simulink model "sim_DF_fixp16_alu"  (R2020b)
settings: Solver=FixedStepDiscrete  StartTime=0.0  StopTime=0.8  FixedStep=DSPBASampleTime  RelTol=1e-3  EnableMultiTasking=on
PreLoadFcn:
  | setup_sim_DF_fixp16_alu;
InitFcn:
  | setup_sim_DF_fixp16_alu;
values from neighbouring files (symbols this model uses):
  ClockFrequency = 100    [setup_DF_fixp16_alu_av.m]    (also in setup_sim_DF_fixp16_alu.m; setup_verify_DF_fixp16_alu.m)
  DSPBASampleTime = FoldingFactor / (ClockFrequency * 1e6)    (= 5e-06)    [setup_DF_fixp16_alu_av.m]    (also in setup_sim_DF_fixp16_alu.m; setup_verify_DF_fixp16_alu.m)
  FoldingFactor = 500    [setup_DF_fixp16_alu_av.m]    (also in setup_sim_DF_fixp16_alu.m; setup_verify_DF_fixp16_alu.m)
  PwmMax = 9375    [setup_sim_DF_fixp16_alu.m]    (also in setup_verify_DF_fixp16_alu.m)
undefined symbols (not defined in the file or in its folder): DiscIntNeverNeededParam, I_max, Position_PI_Limit
libraries: simulink x8, DSPBABase x7, foc_blocks x2
settings Model: Creator=tchau  LastModifiedBy=mhonman
settings DataIOCC: SaveFormat=Array  SaveOutput=off  SignalLogging=off  DSMLogging=off  SaveTime=off  ReturnWorkspaceOutputs=off
settings OptimizationCC: BlockReduction=off  ConditionallyExecuteInputs=off  DefaultParameterBehavior=Inlined  InlineInvariantSignals=on  EfficientFloat2IntCast=on  LifeSpan=inf  SimCompilerOptimization=on
settings DebuggingCC: AlgebraicLoopMsg=error  SolverPrmCheckMsg=warning  SingleTaskRateTransMsg=error  SFUnexpectedBacktrackingDiag=warning  SFNoUnconditionalDefaultTransitionDiag=warning  SFExecutionAtInitializationDiag=none  ArithmeticOperatorsInVariantConditions=warning
settings HardwareCC: ProdBitPerPointer=32  ProdBitPerSizeT=32  ProdBitPerPtrDiffT=32  ProdLargestAtomicFloat=None  ProdIntDivRoundTo=Undefined  ProdEndianess=Unspecified  ProdWordSize=32  ProdHWDeviceType=ASIC/FPGA->ASIC/FPGA  TargetBitPerLong=64  TargetBitPerPointer=64  TargetBitPerSizeT=64  TargetBitPerPtrDiffT=64  TargetLongLongMode=on  TargetIntDivRoundTo=Zero  TargetEndianess=LittleEndian  TargetWordSize=64  TargetHWDeviceType=MATLAB Host  ProdEqTarget=off
settings ModelReferenceCC: PropagateSignalLabelsOutOfModel=off
settings SFSimCC: SimUseLocalCustomCode=off  CustomCodeUndefinedFunction=UseInterfaceOnly
settings RTWCC: RTWUseLocalCustomCode=off
settings CodeAppCC: StateflowObjectComments=on
settings GRTTargetCC: TargetLangStandard=C89/C90 (ANSI)  MatFileLogging=off  SupportNonFinite=off
settings ConfigComp: CovMetricSettings=dw  CovSaveCumulativeToWorkspaceVar=on  CovSaveSingleToWorkspaceVar=on  CovExternalEMLEnable=off

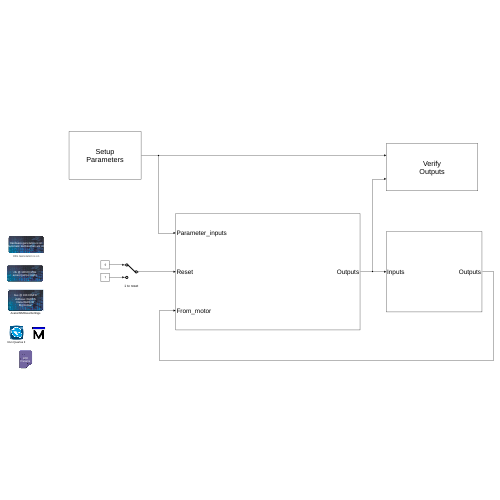
[thumbnail: Simulink's stored preview of the top-level diagram]
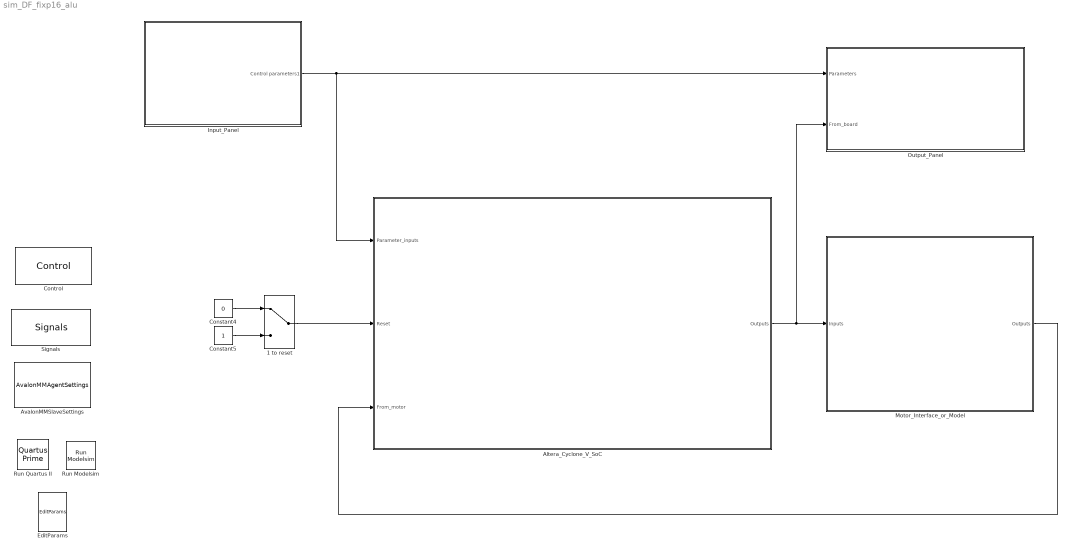
== system sim_DF_fixp16_alu ==
  1 to reset : ManualSwitch
  Altera_Cyclone_V_SoC : Subsystem
  AvalonMMSlaveSettings : DSPBABase/AvalonMMAgentSettings
  Constant4 : Constant  Value=0  OutDataTypeStr=boolean
  Constant5 : Constant  OutDataTypeStr=boolean
  Control : DSPBABase/Control  generate=on  language=VHDL  destination=./rtlmax10  destination_gui=./rtlmax10  make_full_path=off  path_is_relative=on  autotestbench=on  signaldepth=2  coveragetestbench=off  logs=off  spacewidth=2  spacenum=1  addrwidth=6  datawidth=32  dataendian=Big Endian  hierarchicalnames=off  ramThresholdBits=-1  distRamThresholdBits=-1  mlabThresholdBits=-1  hardMultiplierThresholdLuts=-1  version=20090407  errorOnChanMismatch=1  errorOnGPIOMismatch=0  importModelsimResults=0  cycleAccurate=off  reinterpretCastMult=off  paramFile=osim_DF_fixp16_alu_params.xml
      settings: AttributesFormatString=HDL Generation is %<generate>
  EditParams : DSPBABase/EditParams  version=20090407
  Input_Panel : Subsystem
      mask Display: fprintf('Setup\nParameters')
  Motor_Interface_or_Model : Subsystem
  Output_Panel : Subsystem
      mask Display: fprintf('Verify\nOutputs')
  Run Modelsim : DSPBABase/Run Modelsim  version=20090407
  Run Quartus II : DSPBABase/Quartus Prime  version=20090407
  Signals : DSPBABase/Signals  clk=clk  freq=ClockFrequency  margin=0  rst=areset  rstactive=High  bus=bus  enbusclock=off  busfreq=100  bussync=on  version=20090407
  wires:
  Input_Panel/1(Control parameters1) -> Altera_Cyclone_V_SoC/1(Parameter_inputs), Output_Panel/1(Parameters)
  Constant4/1 -> 1 to reset/1
  Constant5/1 -> 1 to reset/2
  1 to reset/1 -> Altera_Cyclone_V_SoC/2(Reset)
  Altera_Cyclone_V_SoC/1(Outputs) -> Motor_Interface_or_Model/1(Inputs), Output_Panel/2(From_board)
  Motor_Interface_or_Model/1(Outputs) -> Altera_Cyclone_V_SoC/3(From_motor)

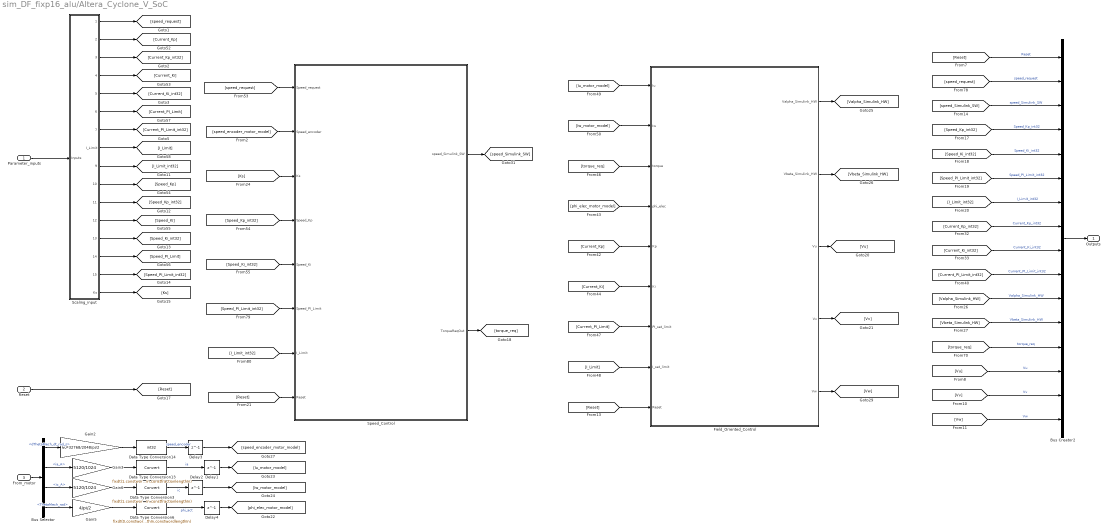
== system sim_DF_fixp16_alu/Altera_Cyclone_V_SoC ==
  Parameter_inputs : Inport
  Reset : Inport  Port=2  PortDimensions=1
  From_motor : Inport  Port=3
  Bus Creator2 : BusCreator  Inputs=16
  Bus Selector : BusSelector  OutputSignals=dThetaMech_dt_rad_s,ia_A,ic_A,ThetaMech_rad
  Data Type Conversion13 : DataTypeConversion  OutDataTypeStr=fixdt(1,constwordlengthIn,constfractionlengthIn)
  Data Type Conversion14 : DataTypeConversion  OutDataTypeStr=int32
  Data Type Conversion3 : DataTypeConversion  OutDataTypeStr=fixdt(1,constwordlengthIn,constfractionlengthIn)
  Data Type Conversion6 : DataTypeConversion  OutDataTypeStr=fixdt(0,constwordlengthIn,constwordlengthIn)
  Delay{1..4} (4 alike) : Delay  DelayLength=1  InitialCondition=0
  Field_Oriented_Control : Subsystem
      mask Display: fprintf('Field-Oriented\nControl')
  Gain2 : Gain  Gain=60*32768/2048/pi/2  OutDataTypeStr=single
  Gain3 : Gain  Gain=5120/1024  OutDataTypeStr=single
  Gain5 : Gain  Gain=4/pi/2  OutDataTypeStr=single
  Gain6 : Gain  Gain=5120/1024  OutDataTypeStr=single
  Scaling_input : Subsystem
  Speed_Control : Subsystem
      mask Display: fprintf('Speed\nControl')
  Outputs : Outport
  wires:
  Speed_Control/2(TorqueReqOut) -> [torque_req]
  Speed_Control/1(speed_Simulink_SW) -> [speed_Simulink_SW]
  [Reset] -> Speed_Control/8(Reset)
  [Ks] -> Speed_Control/3(Ks)
  [speed_Simulink_SW] -> Bus Creator2/3  "speed_Simulink_SW"
  Reset/1 -> [Reset]
  [speed_request] -> Bus Creator2/2  "speed_request"
  Parameter_inputs/1 -> Scaling_input/1(Inputs)
  Scaling_input/1(speed_request) -> [speed_request]
  Scaling_input/2(Current_Kp) -> [Current_Kp]
  Scaling_input/3(Current_Kp_int32) -> [Current_Kp_int32]
  Scaling_input/4(Current_Ki) -> [Current_Ki]
  Scaling_input/5(Current_Ki_int32) -> [Current_Ki_int32]
  Scaling_input/6(Current_PI_Limit) -> [Current_PI_Limit]
  Scaling_input/7(Current_PI_Limit_int32) -> [Current_PI_Limit_int32]
  Scaling_input/8(I_Limit) -> [I_Limit]
  Scaling_input/9(I_Limit_int32) -> [I_Limit_int32]
  Scaling_input/10(Speed_Kp) -> [Speed_Kp]
  Scaling_input/11(Speed_Kp_int32) -> [Speed_Kp_int32]
  Scaling_input/12(Speed_Ki) -> [Speed_Ki]
  Scaling_input/13(Speed_Ki_int32) -> [Speed_Ki_int32]
  Scaling_input/14(Speed_PI_Limit) -> [Speed_PI_Limit]
  Scaling_input/15(Speed_PI_Limit_int32) -> [Speed_PI_Limit_int32]
  Scaling_input/16(Ks) -> [Ks]
  [speed_request] -> Speed_Control/1(Speed_request)
  [Speed_Kp_int32] -> Speed_Control/4(Speed_Kp)
  [Speed_Ki_int32] -> Speed_Control/5(Speed_Ki)
  [Speed_PI_Limit_int32] -> Speed_Control/6(Speed_PI_Limit)
  [I_Limit_int32] -> Speed_Control/7(I_Limit)
  [Speed_Kp_int32] -> Bus Creator2/4  "Speed_Kp_int32"
  [Speed_Ki_int32] -> Bus Creator2/5  "Speed_Ki_int32"
  [Speed_PI_Limit_int32] -> Bus Creator2/6  "Speed_PI_Limit_int32"
  [I_Limit_int32] -> Bus Creator2/7  "I_Limit_int32"
  [Current_Kp_int32] -> Bus Creator2/8  "Current_Kp_int32"
  [Current_Ki_int32] -> Bus Creator2/9  "Current_Ki_int32"
  [Current_PI_Limit_int32] -> Bus Creator2/10  "Current_PI_Limit_int32"
  [Reset] -> Bus Creator2/1  "Reset"
  Bus Creator2/1 -> Outputs/1
  [Valpha_Simulink_HW] -> Bus Creator2/11  "Valpha_Simulink_HW"
  [Vbeta_Simulink_HW] -> Bus Creator2/12  "Vbeta_Simulink_HW"
  [torque_req] -> Bus Creator2/13  "torque_req"
  [Iu_motor_model] -> Field_Oriented_Control/1(Iu)
  [Iw_motor_model] -> Field_Oriented_Control/2(Iw)
  [torque_req] -> Field_Oriented_Control/3(torque)
  [phi_elec_motor_model] -> Field_Oriented_Control/4(phi_elec)
  [Current_Kp] -> Field_Oriented_Control/5(Kp)
  [Current_Ki] -> Field_Oriented_Control/6(Ki)
  [Current_PI_Limit] -> Field_Oriented_Control/7(PI_sat_limit)
  [I_Limit] -> Field_Oriented_Control/8(I_sat_limit)
  [Reset] -> Field_Oriented_Control/9(Reset)
  Field_Oriented_Control/1(Valpha_Simulink_HW) -> [Valpha_Simulink_HW]
  Field_Oriented_Control/2(Vbeta_Simulink_HW) -> [Vbeta_Simulink_HW]
  Field_Oriented_Control/3(Vu) -> [Vu]
  From_motor/1 -> Bus Selector/1
  [speed_encoder_motor_model] -> Speed_Control/2(Speed_encoder)
  Delay1/1 -> [Iu_motor_model]
  Delay2/1 -> [Iw_motor_model]
  Delay4/1 -> [phi_elec_motor_model]
  Bus Selector/3 -> Gain6/1  "<ic_A>"
  Delay3/1 -> [speed_encoder_motor_model]
  Bus Selector/1 -> Gain2/1  "<dThetaMech_dt_rad_s>"
  Bus Selector/4 -> Gain5/1  "<ThetaMech_rad>"
  Bus Selector/2 -> Gain3/1  "<ia_A>"
  [Vu] -> Bus Creator2/14  "Vu"
  [Vv] -> Bus Creator2/15  "Vv"
  [Vw] -> Bus Creator2/16  "Vw"
  Gain2/1 -> Data Type Conversion14/1
  Data Type Conversion14/1 -> Delay3/1  "speed_encoder"
  Gain5/1 -> Data Type Conversion6/1
  Data Type Conversion6/1 -> Delay4/1  "phi_act"
  Gain3/1 -> Data Type Conversion13/1
  Data Type Conversion13/1 -> Delay1/1  "ia"
  Gain6/1 -> Data Type Conversion3/1
  Data Type Conversion3/1 -> Delay2/1  "ic"
  Field_Oriented_Control/4(Vv) -> [Vv]
  Field_Oriented_Control/5(Vw) -> [Vw]

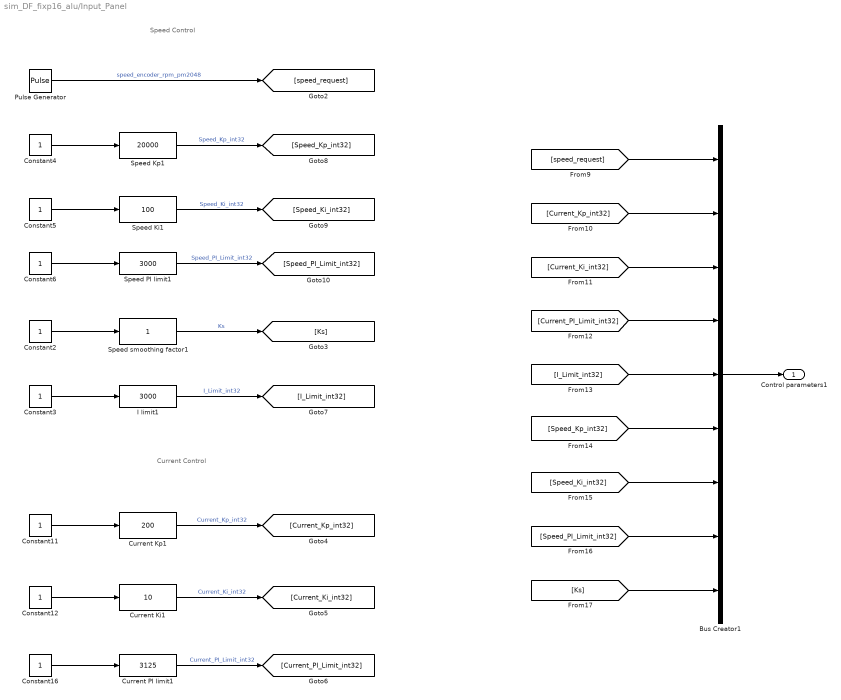
== system sim_DF_fixp16_alu/Input_Panel ==
  note: Speed Control
  note: Current Control
  Bus Creator1 : BusCreator  Inputs=9
  Constant{3..6,11..12,16} (7 alike) : Constant  OutDataTypeStr=int32
  Constant2 : Constant  OutDataTypeStr=fixdt(0,16,15)
  Current Ki1 : simulink/Math Operations/Slider Gain  gain=10  low=0  high=100
  Current Kp1 : simulink/Math Operations/Slider Gain  gain=200  low=0  high=1000
  Current PI limit1 : simulink/Math Operations/Slider Gain  gain=3125  low=0  high=10000
  I limit1 : simulink/Math Operations/Slider Gain  gain=3000  low=0  high=10000
  Pulse Generator : DiscretePulseGenerator  Amplitude=50  Period=ClockFrequency * 1e6 / FoldingFactor * 5  PulseWidth=ClockFrequency * 1e6 / FoldingFactor * 2.5  SampleTime=DSPBASampleTime
  Speed Ki1 : simulink/Math Operations/Slider Gain  gain=100  low=0  high=1000
  Speed Kp1 : simulink/Math Operations/Slider Gain  gain=20000  low=0  high=100000
  Speed PI limit1 : simulink/Math Operations/Slider Gain  gain=3000  low=0  high=10000
  Speed smoothing factor1 : simulink/Math Operations/Slider Gain  gain=1  low=0  high=1
  Control parameters1 : Outport
  wires:
  Pulse Generator/1 -> [speed_request]  "speed_encoder_rpm_pm2048"
  [Ks] -> Bus Creator1/9
  [Speed_PI_Limit_int32] -> Bus Creator1/8
  [Speed_Ki_int32] -> Bus Creator1/7
  [Speed_Kp_int32] -> Bus Creator1/6
  [I_Limit_int32] -> Bus Creator1/5
  [Current_PI_Limit_int32] -> Bus Creator1/4
  [Current_Ki_int32] -> Bus Creator1/3
  [Current_Kp_int32] -> Bus Creator1/2
  [speed_request] -> Bus Creator1/1
  Bus Creator1/1 -> Control parameters1/1
  Constant2/1 -> Speed smoothing factor1/1
  Speed smoothing factor1/1 -> [Ks]  "Ks"
  Speed Kp1/1 -> [Speed_Kp_int32]  "Speed_Kp_int32"
  Speed Ki1/1 -> [Speed_Ki_int32]  "Speed_Ki_int32"
  Speed PI limit1/1 -> [Speed_PI_Limit_int32]  "Speed_PI_Limit_int32"
  Constant4/1 -> Speed Kp1/1
  Constant5/1 -> Speed Ki1/1
  Constant6/1 -> Speed PI limit1/1
  Current Kp1/1 -> [Current_Kp_int32]  "Current_Kp_int32"
  Current Ki1/1 -> [Current_Ki_int32]  "Current_Ki_int32"
  Current PI limit1/1 -> [Current_PI_Limit_int32]  "Current_PI_Limit_int32"
  I limit1/1 -> [I_Limit_int32]  "I_Limit_int32"
  Constant11/1 -> Current Kp1/1
  Constant12/1 -> Current Ki1/1
  Constant16/1 -> Current PI limit1/1
  Constant3/1 -> I limit1/1

== system sim_DF_fixp16_alu/Motor_Interface_or_Model ==
  Inputs : Inport
  Bus Selector : BusSelector  OutputSignals=Vu,Vv,Vw
  Constant1 : Constant  Value=0  OutDataTypeStr=Inherit: Inherit via back propagation
  Data Type Conversion1 : DataTypeConversion  OutDataTypeStr=double
  Data Type Conversion4 : DataTypeConversion  OutDataTypeStr=double
  Data Type Conversion5 : DataTypeConversion  OutDataTypeStr=double
  MotorContinuousTime4 : Subsystem  mask(AlteraPMSM){R_ohm=21.4/2, L_H=37.5e-3/2, Ke_Vs_rad=0.85/sqrt(2), Kt_Nm_A=0.85/sqrt(2), PolePairs_int=4, J_kgm2=0.33e-4}
      mask prompts: R_ohm "Phase resistance [Ohm]"; L_H "Phase inductance [H]"; Ke_Vs_rad "Back-emf constant kE, based on peak phase values [Vs/rad]"; Kt_Nm_A "Motor torque constant kT, based on peak phase values [Nm/A]"; PolePairs_int "Number of pole pairs (0.5*n poles)  [integer]"; J_kgm2 "Mechanical inertia [kgm^2]"
      mask help: Altera motor model
      mask Display: fprintf('Motor\nModel')
  Outputs : Outport
  wires:
  Constant1/1 -> MotorContinuousTime4/4(Load Torque [Nm])
  Inputs/1 -> Bus Selector/1
  Data Type Conversion4/1 -> MotorContinuousTime4/1(Va_V)
  Data Type Conversion1/1 -> MotorContinuousTime4/2(Vb_V)
  Data Type Conversion5/1 -> MotorContinuousTime4/3(Vc_V)
  Bus Selector/1 -> Data Type Conversion4/1  "<Vu>"
  Bus Selector/2 -> Data Type Conversion1/1  "<Vv>"
  Bus Selector/3 -> Data Type Conversion5/1  "<Vw>"
  MotorContinuousTime4/1(OutputBus) -> Outputs/1

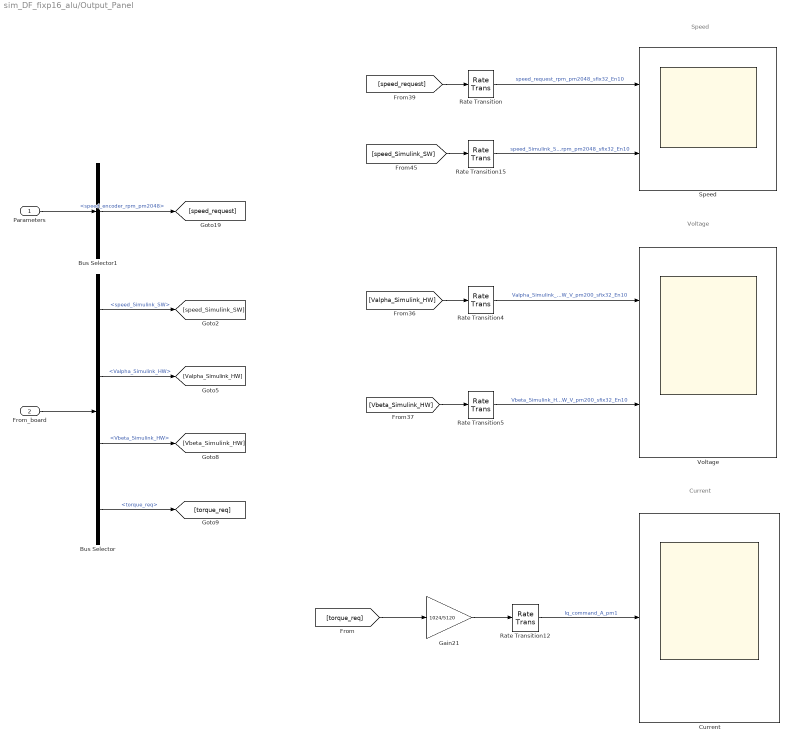
== system sim_DF_fixp16_alu/Output_Panel ==
  note: Speed
  note: Voltage
  note: Current
  Parameters : Inport
  From_board : Inport  Port=2
  Bus Selector : BusSelector  OutputSignals=speed_Simulink_SW,Valpha_Simulink_HW,Vbeta_Simulink_HW,torque_req
  Bus Selector1 : BusSelector  OutputSignals=speed_encoder_rpm_pm2048
  Current : Scope
  Gain21 : Gain  Gain=1024/5120
  Rate Transition{,4..5,12,15} (5 alike) : RateTransition
  Speed : Scope  NumInputPorts=2
  Voltage : Scope  NumInputPorts=2
  wires:
  Rate Transition4/1 -> Voltage/1  "Valpha_Simulink_HW_V_pm200_sfix32_En10"
  Rate Transition5/1 -> Voltage/2  "Vbeta_Simulink_HW_V_pm200_sfix32_En10"
  Rate Transition/1 -> Speed/1  "speed_request_rpm_pm2048_sfix32_En10"
  [speed_request] -> Rate Transition/1
  Rate Transition15/1 -> Speed/2  "speed_Simulink_SW_rpm_pm2048_sfix32_En10"
  [speed_Simulink_SW] -> Rate Transition15/1
  [torque_req] -> Gain21/1
  Rate Transition12/1 -> Current/1  "Iq_command_A_pm1"
  Gain21/1 -> Rate Transition12/1
  [Valpha_Simulink_HW] -> Rate Transition4/1
  [Vbeta_Simulink_HW] -> Rate Transition5/1
  From_board/1 -> Bus Selector/1
  Parameters/1 -> Bus Selector1/1
  Bus Selector1/1 -> [speed_request]  "<speed_encoder_rpm_pm2048>"
  Bus Selector/1 -> [speed_Simulink_SW]  "<speed_Simulink_SW>"
  Bus Selector/2 -> [Valpha_Simulink_HW]  "<Valpha_Simulink_HW>"
  Bus Selector/3 -> [Vbeta_Simulink_HW]  "<Vbeta_Simulink_HW>"
  Bus Selector/4 -> [torque_req]  "<torque_req>"

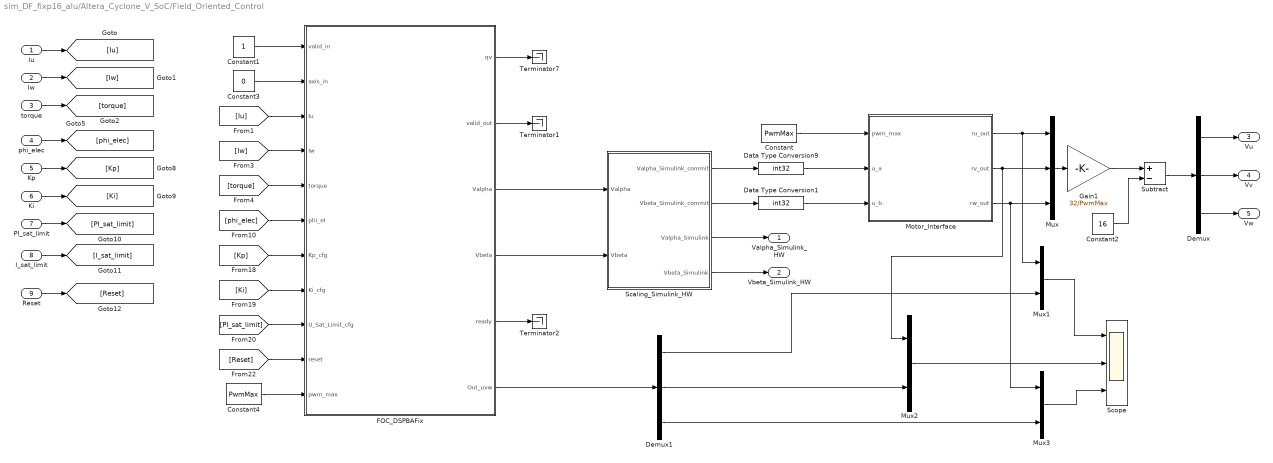
== system sim_DF_fixp16_alu/Altera_Cyclone_V_SoC/Field_Oriented_Control ==
  Iu : Inport
  Iw : Inport  Port=2
  torque : Inport  Port=3
  phi_elec : Inport  Port=4
  Kp : Inport  Port=5
  Ki : Inport  Port=6
  PI_sat_limit : Inport  Port=7
  I_sat_limit : Inport  Port=8
  Reset : Inport  Port=9
  Constant : Constant  Value=PwmMax  OutDataTypeStr=uint16
  Constant1 : Constant  OutDataTypeStr=boolean
  Constant2 : Constant  Value=16  OutDataTypeStr=int32
  Constant3 : Constant  Value=0  OutDataTypeStr=uint32
  Constant4 : Constant  Value=PwmMax  OutDataTypeStr=uint16
  Data Type Conversion1 : DataTypeConversion  OutDataTypeStr=int32
  Data Type Conversion9 : DataTypeConversion  OutDataTypeStr=int32
  Demux : Demux  Outputs=3
  Demux1 : Demux  Outputs=3
  FOC_DSPBAFix : Subsystem
  Gain1 : Gain  Gain=32/PwmMax
  Motor_Interface : MATLAB Function  TreatAsAtomicUnit=on
  Mux : Mux  Inputs=3
  Mux1 : Mux  Inputs=2
  Mux2 : Mux  Inputs=2
  Mux3 : Mux  Inputs=2
  Scaling_Simulink_HW : Subsystem
  Scope : Scope  NumInputPorts=3
  Subtract : Sum  Inputs=+-
  Terminator1 : Terminator
  Terminator2 : Terminator
  Terminator7 : Terminator
  Valpha_Simulink_HW : Outport
  Vbeta_Simulink_HW : Outport  Port=2
  Vu : Outport  Port=3
  Vv : Outport  Port=4
  Vw : Outport  Port=5
  wires:
  FOC_DSPBAFix/3(Valpha) -> Scaling_Simulink_HW/1(Valpha)
  FOC_DSPBAFix/4(Vbeta) -> Scaling_Simulink_HW/2(Vbeta)
  Scaling_Simulink_HW/3(Valpha_Simulink) -> Valpha_Simulink_HW/1
  Scaling_Simulink_HW/4(Vbeta_Simulink) -> Vbeta_Simulink_HW/1
  Iu/1 -> [Iu]
  [Iu] -> FOC_DSPBAFix/3(Iu)
  [Iw] -> FOC_DSPBAFix/4(Iw)
  Iw/1 -> [Iw]
  torque/1 -> [torque]
  [torque] -> FOC_DSPBAFix/5(torque)
  phi_elec/1 -> [phi_elec]
  [phi_elec] -> FOC_DSPBAFix/6(phi_el)
  Kp/1 -> [Kp]
  Ki/1 -> [Ki]
  PI_sat_limit/1 -> [PI_sat_limit]
  I_sat_limit/1 -> [I_sat_limit]
  Reset/1 -> [Reset]
  [Kp] -> FOC_DSPBAFix/7(Kp_cfg)
  [Ki] -> FOC_DSPBAFix/8(Ki_cfg)
  [PI_sat_limit] -> FOC_DSPBAFix/9(U_Sat_Limit_cfg)
  [Reset] -> FOC_DSPBAFix/10(reset)
  Scaling_Simulink_HW/1(Valpha_Simulink_commit) -> Data Type Conversion9/1
  Scaling_Simulink_HW/2(Vbeta_Simulink_commit) -> Data Type Conversion1/1
  Constant1/1 -> FOC_DSPBAFix/1(valid_in)
  Constant3/1 -> FOC_DSPBAFix/2(axis_in)
  FOC_DSPBAFix/1(qv) -> Terminator7/1
  FOC_DSPBAFix/2(valid_out) -> Terminator1/1
  FOC_DSPBAFix/5(ready) -> Terminator2/1
  Constant4/1 -> FOC_DSPBAFix/11(pwm_max)
  FOC_DSPBAFix/6(Out_uvw) -> Demux1/1
  Mux2/1 -> Scope/2
  Mux1/1 -> Scope/1
  Demux1/3 -> Mux3/2
  Demux1/2 -> Mux2/2
  Mux3/1 -> Scope/3
  Demux1/1 -> Mux1/2
  Demux/2 -> Vv/1
  Mux/1 -> Gain1/1
  Demux/3 -> Vw/1
  Constant2/1 -> Subtract/2
  Motor_Interface/3(rw_out) -> Mux3/1, Mux/3
  Demux/1 -> Vu/1
  Motor_Interface/1(ru_out) -> Mux1/1, Mux/1
  Subtract/1 -> Demux/1
  Motor_Interface/2(rv_out) -> Mux2/1, Mux/2
  Gain1/1 -> Subtract/1
  Data Type Conversion1/1 -> Motor_Interface/3(u_b)
  Data Type Conversion9/1 -> Motor_Interface/2(u_a)
  Constant/1 -> Motor_Interface/1(pwm_max)

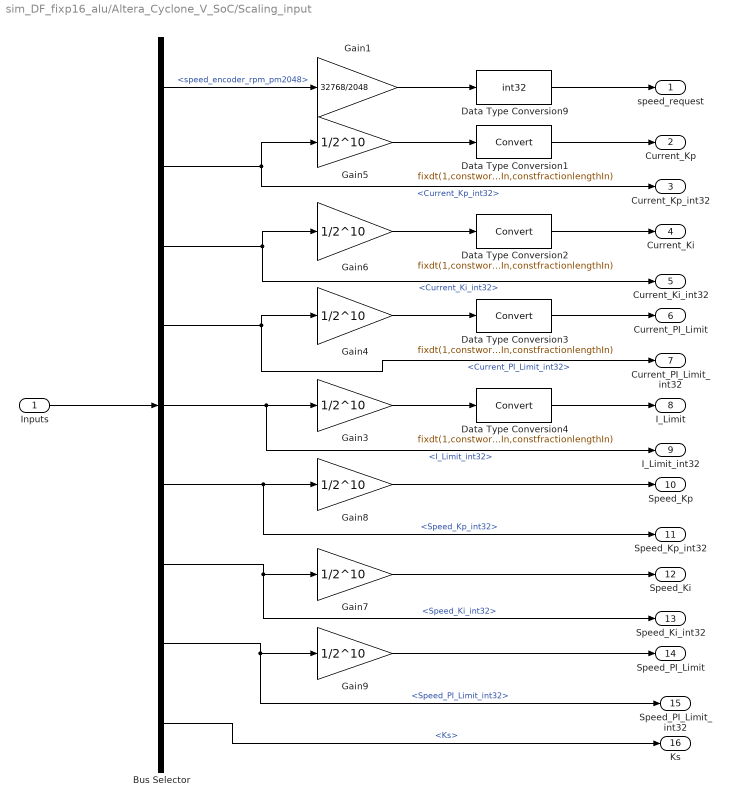
== system sim_DF_fixp16_alu/Altera_Cyclone_V_SoC/Scaling_input ==
  Inputs : Inport
  Bus Selector : BusSelector  OutputSignals=speed_encoder_rpm_pm2048,Current_Kp_int32,Current_Ki_int32,Current_PI_Limit_int32,I_Limit_int32,Speed_Kp_int32,Speed_Ki_int32,Speed_PI_Limit_int32,Ks
  Data Type Conversion{1..4} (4 alike) : DataTypeConversion  OutDataTypeStr=fixdt(1,constwordlengthIn,constfractionlengthIn)
  Data Type Conversion9 : DataTypeConversion  OutDataTypeStr=int32
  Gain1 : Gain  Gain=32768/2048
  Gain{3..9} (7 alike) : Gain  Gain=1/2^10  OutDataTypeStr=single
  speed_request : Outport
  Current_Kp : Outport  Port=2
  Current_Kp_int32 : Outport  Port=3
  Current_Ki : Outport  Port=4
  Current_Ki_int32 : Outport  Port=5
  Current_PI_Limit : Outport  Port=6
  Current_PI_Limit_int32 : Outport  Port=7
  I_Limit : Outport  Port=8
  I_Limit_int32 : Outport  Port=9
  Speed_Kp : Outport  Port=10
  Speed_Kp_int32 : Outport  Port=11
  Speed_Ki : Outport  Port=12
  Speed_Ki_int32 : Outport  Port=13
  Speed_PI_Limit : Outport  Port=14
  Speed_PI_Limit_int32 : Outport  Port=15
  Ks : Outport  Port=16
  wires:
  Bus Selector/7 -> Speed_Ki_int32/1, Gain7/1  "<Speed_Ki_int32>"
  Gain8/1 -> Speed_Kp/1
  Bus Selector/8 -> Speed_PI_Limit_int32/1, Gain9/1  "<Speed_PI_Limit_int32>"
  Bus Selector/6 -> Speed_Kp_int32/1, Gain8/1  "<Speed_Kp_int32>"
  Bus Selector/9 -> Ks/1  "<Ks>"
  Data Type Conversion3/1 -> Current_PI_Limit/1
  Bus Selector/2 -> Current_Kp_int32/1, Gain5/1  "<Current_Kp_int32>"
  Bus Selector/1 -> Gain1/1  "<speed_encoder_rpm_pm2048>"
  Bus Selector/3 -> Current_Ki_int32/1, Gain6/1  "<Current_Ki_int32>"
  Gain9/1 -> Speed_PI_Limit/1
  Data Type Conversion2/1 -> Current_Ki/1
  Inputs/1 -> Bus Selector/1
  Data Type Conversion1/1 -> Current_Kp/1
  Data Type Conversion4/1 -> I_Limit/1
  Gain5/1 -> Data Type Conversion1/1
  Gain3/1 -> Data Type Conversion4/1
  Gain6/1 -> Data Type Conversion2/1
  Gain7/1 -> Speed_Ki/1
  Bus Selector/5 -> I_Limit_int32/1, Gain3/1  "<I_Limit_int32>"
  Bus Selector/4 -> Current_PI_Limit_int32/1, Gain4/1  "<Current_PI_Limit_int32>"
  Gain4/1 -> Data Type Conversion3/1
  Gain1/1 -> Data Type Conversion9/1
  Data Type Conversion9/1 -> speed_request/1

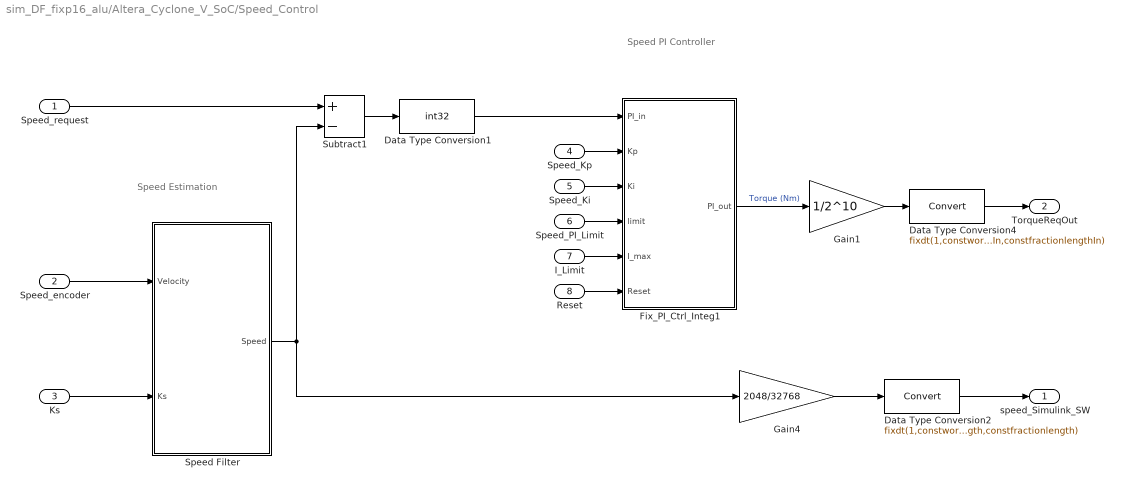
== system sim_DF_fixp16_alu/Altera_Cyclone_V_SoC/Speed_Control ==
  note: Speed
      | PI Controller
  note: Speed Estimation
  Speed_request : Inport  PortDimensions=1
  Speed_encoder : Inport  Port=2  PortDimensions=1
  Ks : Inport  Port=3  PortDimensions=1
  Speed_Kp : Inport  Port=4  PortDimensions=1
  Speed_Ki : Inport  Port=5  PortDimensions=1
  Speed_PI_Limit : Inport  Port=6  PortDimensions=1
  I_Limit : Inport  Port=7  PortDimensions=1
  Reset : Inport  Port=8  PortDimensions=1
  Data Type Conversion1 : DataTypeConversion  OutDataTypeStr=int32
  Data Type Conversion2 : DataTypeConversion  OutDataTypeStr=fixdt(1,constwordlength,constfractionlength)
  Data Type Conversion4 : DataTypeConversion  OutDataTypeStr=fixdt(1,constwordlengthIn,constfractionlengthIn)
  Fix_PI_Ctrl_Integ1 : Subsystem
  Gain1 : Gain  Gain=1/2^10
  Gain4 : Gain  Gain=2048/32768  OutDataTypeStr=single
  Speed Filter : Subsystem
  Subtract1 : Sum  Inputs=+-
  speed_Simulink_SW : Outport  PortDimensions=1
  TorqueReqOut : Outport  Port=2  PortDimensions=1
  wires:
  Data Type Conversion4/1 -> TorqueReqOut/1
  Speed Filter/1(Speed) -> Subtract1/2, Gain4/1
  I_Limit/1 -> Fix_PI_Ctrl_Integ1/5(I_max)
  Speed_PI_Limit/1 -> Fix_PI_Ctrl_Integ1/4(limit)
  Speed_Ki/1 -> Fix_PI_Ctrl_Integ1/3(Ki)
  Speed_Kp/1 -> Fix_PI_Ctrl_Integ1/2(Kp)
  Subtract1/1 -> Data Type Conversion1/1
  Fix_PI_Ctrl_Integ1/1(PI_out) -> Gain1/1  "Torque (Nm)"
  Data Type Conversion1/1 -> Fix_PI_Ctrl_Integ1/1(PI_in)
  Gain1/1 -> Data Type Conversion4/1
  Gain4/1 -> Data Type Conversion2/1
  Data Type Conversion2/1 -> speed_Simulink_SW/1
  Ks/1 -> Speed Filter/2(Ks)
  Reset/1 -> Fix_PI_Ctrl_Integ1/6(Reset)
  Speed_encoder/1 -> Speed Filter/1(Velocity)
  Speed_request/1 -> Subtract1/1

== system sim_DF_fixp16_alu/Motor_Interface_or_Model/MotorContinuousTime4 ==
  Va_V : Inport
  Vb_V : Inport  Port=2
  Vc_V : Inport  Port=3
  Load Torque [Nm] : Inport  Port=4
  Bus Creator1 : BusCreator  Inputs=12
  Motor electromagnetic : Subsystem
  Motor inertia : Subsystem  mask(Inertia){J_kgm2=J_kgm2}
      mask prompts: J_kgm2 "Inertia [kgm^2]"
      mask help:
      | Mechanical inertia with two attachment points A and B.
      | Torque is applied to the inertia from side A and side B.
      | The combined torque acting on the inertia produces acceleration,
      | velocity and displacement. Velocity and displacement are output as these
      | are the states of the system.
  OutputBus : Outport
  wires:
  Motor inertia/2(Theta_rad) -> Bus Creator1/11, Motor electromagnetic/4(ThetaMech_rad)  "ThetaMech_rad"
  Motor inertia/1(dTheta_dt_rad_s) -> Bus Creator1/12, Motor electromagnetic/5(dThetaMech_dt_rad_s)  "dThetaMech_dt_rad_s"
  Motor electromagnetic/1(ia_A) -> Bus Creator1/1  "ia_A"
  Load Torque [Nm]/1 -> Motor inertia/2(TB_Nm)
  Vb_V/1 -> Motor electromagnetic/2(Vb_V)
  Va_V/1 -> Motor electromagnetic/1(Va_V)
  Vc_V/1 -> Motor electromagnetic/3(Vc_V)
  Motor electromagnetic/2(ib_A) -> Bus Creator1/2  "ib_A"
  Motor electromagnetic/3(ic_A) -> Bus Creator1/3  "ic_A"
  Motor electromagnetic/4(T_Nm) -> Motor inertia/1(TA_Nm), Bus Creator1/4  "T_Nm"
  Motor electromagnetic/5(id_A) -> Bus Creator1/5  "id_A"
  Motor electromagnetic/6(iq_A) -> Bus Creator1/6  "iq_A"
  Motor electromagnetic/7(vd_V) -> Bus Creator1/7  "vd_V"
  Motor electromagnetic/8(vq_V) -> Bus Creator1/8  "vq_V"
  Motor electromagnetic/9(did_dt_A_s) -> Bus Creator1/9  "did_dt_A_s"
  Motor electromagnetic/10(diq_dt_A_s) -> Bus Creator1/10  "diq_dt_A_s"
  Bus Creator1/1 -> OutputBus/1

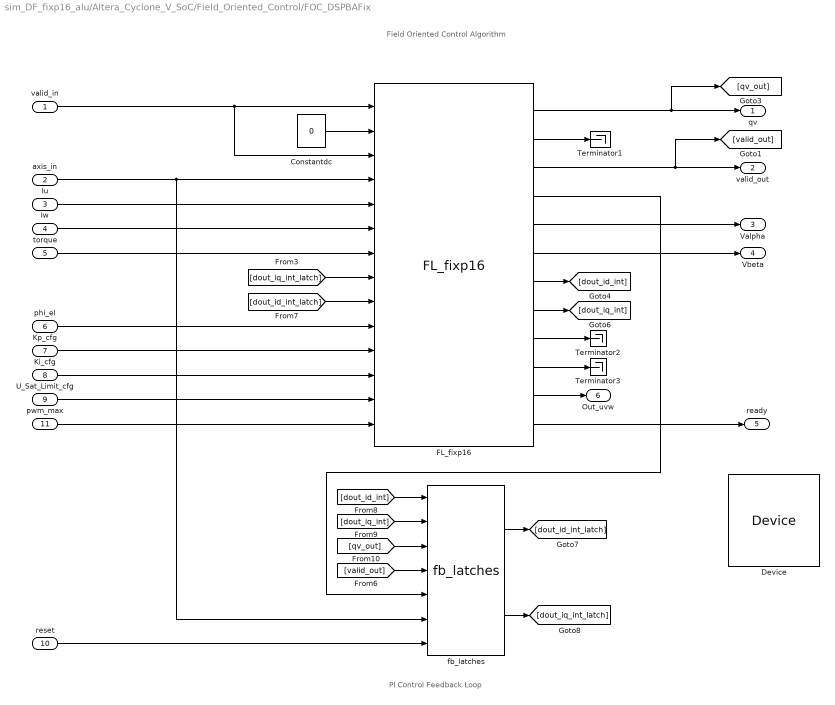
== system sim_DF_fixp16_alu/Altera_Cyclone_V_SoC/Field_Oriented_Control/FOC_DSPBAFix ==
  note: PI Control Feedback Loop
  note: Field Oriented Control Algorithm
  valid_in : Inport
  axis_in : Inport  Port=2
  Iu : Inport  Port=3
  Iw : Inport  Port=4
  torque : Inport  Port=5
  phi_el : Inport  Port=6
  Kp_cfg : Inport  Port=7
  Ki_cfg : Inport  Port=8
  U_Sat_Limit_cfg : Inport  Port=9
  reset : Inport  Port=10
  pwm_max : Inport  Port=11
  Constantdc : Constant  Value=0  OutDataTypeStr=uint8  SampleTime=DSPBASampleTime
  Device : DSPBABase/Device  family=MAX 10  deviceMember=Stratix V GX  stratix4device=Stratix IV E  hardcopy4device=HardCopy IV E  stratix5device=Stratix V GX  device=AUTO  speed=6  stratixSpeed=-5  stratix2Speed=-3  stratix3Speed=-2  stratix4gxSpeed=-2  stratix4gtSpeed=-1  cyclone2Speed=-6  cyclone3Speed=-7  arria2Speed=-4  cyclone4eSpeed=-8  stratix5Speed=-3  arria5Speed=-4  arriaSpeed=-6  cyclone3lsSpeed=-7  cyclone5Speed=-6  arria2gzSpeed=-3  nightFurySpeed=-2  ecp2Speed=-7  hardcopycompat=off  version=20140217  max10flashmode=off  max10nomeminit=off
  FL_fixp16 : foc_blocks/FL_fixp16  SystemSampleTime=-1  VariantActivationTime=update diagram  Latency=0  AutoFrameSizeCalculation=off
      link override ChannelOut1: latency=20
      settings: SourceProductName=FOC Blocks
  Terminator1 : Terminator
  Terminator2 : Terminator
  Terminator3 : Terminator
  fb_latches : foc_blocks/fb_latches  SystemSampleTime=-1  VariantActivationTime=update diagram  Latency=0  AutoFrameSizeCalculation=off
      link override GPOut1: latency=1
      link override GPOut2: latency=1
      settings: SourceProductName=FOC Blocks
  qv : Outport
  valid_out : Outport  Port=2
  Valpha : Outport  Port=3
  Vbeta : Outport  Port=4
  ready : Outport  Port=5
  Out_uvw : Outport  Port=6
  wires:
  reset/1 -> fb_latches/7
  [valid_out] -> fb_latches/4
  fb_latches/2 -> [dout_iq_int_latch]
  fb_latches/1 -> [dout_id_int_latch]
  [dout_iq_int] -> fb_latches/2
  [dout_id_int] -> fb_latches/1
  [qv_out] -> fb_latches/3
  FL_fixp16/4 -> fb_latches/5
  axis_in/1 -> fb_latches/6, FL_fixp16/4
  U_Sat_Limit_cfg/1 -> FL_fixp16/13
  Ki_cfg/1 -> FL_fixp16/12
  Kp_cfg/1 -> FL_fixp16/11
  phi_el/1 -> FL_fixp16/10
  torque/1 -> FL_fixp16/7
  Iw/1 -> FL_fixp16/6
  Iu/1 -> FL_fixp16/5
  valid_in/1 -> FL_fixp16/3, FL_fixp16/1
  FL_fixp16/2 -> Terminator1/1
  [dout_id_int_latch] -> FL_fixp16/9
  [dout_iq_int_latch] -> FL_fixp16/8
  FL_fixp16/7 -> [dout_id_int]
  FL_fixp16/8 -> [dout_iq_int]
  Constantdc/1 -> FL_fixp16/2
  FL_fixp16/6 -> Vbeta/1
  FL_fixp16/3 -> [valid_out], valid_out/1
  FL_fixp16/1 -> [qv_out], qv/1
  FL_fixp16/5 -> Valpha/1
  FL_fixp16/11 -> Out_uvw/1
  pwm_max/1 -> FL_fixp16/14
  FL_fixp16/12 -> ready/1
  FL_fixp16/9 -> Terminator2/1
  FL_fixp16/10 -> Terminator3/1

== system sim_DF_fixp16_alu/Altera_Cyclone_V_SoC/Field_Oriented_Control/Scaling_Simulink_HW ==
  Valpha : Inport
  Vbeta : Inport  Port=2
  Gain12 : Gain  Gain=190/1563
  Gain13 : Gain  Gain=190/1563
  Gain14 : Gain  Gain=2^10
  Gain16 : Gain  Gain=2^10
  Valpha_Simulink_commit : Outport
  Vbeta_Simulink_commit : Outport  Port=2
  Valpha_Simulink : Outport  Port=3
  Vbeta_Simulink : Outport  Port=4
  wires:
  Gain14/1 -> Gain12/1, Valpha_Simulink_commit/1
  Valpha/1 -> Gain14/1
  Gain16/1 -> Gain13/1, Vbeta_Simulink_commit/1
  Vbeta/1 -> Gain16/1
  Gain13/1 -> Vbeta_Simulink/1
  Gain12/1 -> Valpha_Simulink/1

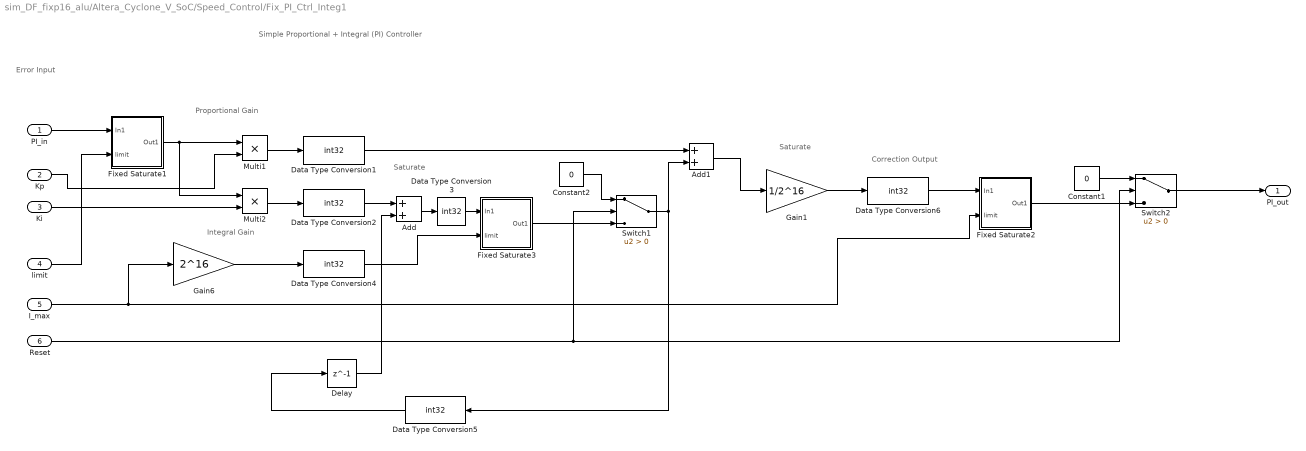
== system sim_DF_fixp16_alu/Altera_Cyclone_V_SoC/Speed_Control/Fix_PI_Ctrl_Integ1 ==
  note: Simple Proportional + Integral (PI) Controller
  note: Error Input
  note: Proportional Gain
  note: Integral Gain
  note: Saturate
  note: Saturate
  note: Correction Output
  PI_in : Inport
  Kp : Inport  Port=2
  Ki : Inport  Port=3
  limit : Inport  Port=4
  I_max : Inport  Port=5
  Reset : Inport  Port=6
  Add : Sum
  Add1 : Sum
  Constant1 : Constant  Value=0  OutDataTypeStr=Inherit: Inherit via back propagation
  Constant2 : Constant  Value=0  OutDataTypeStr=Inherit: Inherit via back propagation
  Data Type Conversion{1..6} (6 alike) : DataTypeConversion  OutDataTypeStr=int32
  Delay : Delay  DelayLength=1  InitialCondition=0
  Fixed Saturate1 : Subsystem
  Fixed Saturate2 : Subsystem
  Fixed Saturate3 : Subsystem
  Gain1 : Gain  Gain=1/2^16
  Gain6 : Gain  Gain=2^16
  Multi1 : Product  Inputs=**  RndMeth=Zero  SaturateOnIntegerOverflow=on
  Multi2 : Product  Inputs=**  RndMeth=Zero  SaturateOnIntegerOverflow=on
  Switch1 : Switch  Criteria=u2 > Threshold
  Switch2 : Switch  Criteria=u2 > Threshold
  PI_out : Outport
  wires:
  Ki/1 -> Multi2/2
  Kp/1 -> Multi1/2
  I_max/1 -> Fixed Saturate2/2(limit), Gain6/1
  Multi2/1 -> Data Type Conversion2/1
  Multi1/1 -> Data Type Conversion1/1
  Add1/1 -> Gain1/1
  Add/1 -> Data Type Conversion3/1
  Delay/1 -> Add/2
  Fixed Saturate1/1(Out1) -> Multi1/1, Multi2/1
  PI_in/1 -> Fixed Saturate1/1(In1)
  limit/1 -> Fixed Saturate1/2(limit)
  Gain6/1 -> Data Type Conversion4/1
  Gain1/1 -> Data Type Conversion6/1
  Data Type Conversion4/1 -> Fixed Saturate3/2(limit)
  Data Type Conversion1/1 -> Add1/1
  Data Type Conversion2/1 -> Add/1
  Data Type Conversion3/1 -> Fixed Saturate3/1(In1)
  Data Type Conversion5/1 -> Delay/1
  Data Type Conversion6/1 -> Fixed Saturate2/1(In1)
  Fixed Saturate2/1(Out1) -> Switch2/3
  Switch2/1 -> PI_out/1
  Reset/1 -> Switch1/2, Switch2/2
  Constant1/1 -> Switch2/1
  Constant2/1 -> Switch1/1
  Fixed Saturate3/1(Out1) -> Switch1/3
  Switch1/1 -> Data Type Conversion5/1, Add1/2

== system sim_DF_fixp16_alu/Altera_Cyclone_V_SoC/Speed_Control/Speed Filter ==
  Velocity : Inport
  Ks : Inport  Port=2
  Add : Sum  Inputs=-+
  Constant6 : Constant  OutDataTypeStr=Inherit: Inherit via back propagation
  Data Type Conversion1 : DataTypeConversion  OutDataTypeStr=int32
  Data Type Conversion4 : DataTypeConversion  OutDataTypeStr=int32
  Delay1 : Delay  DelayLength=1  InitialCondition=0
  Multi1 : Product  Inputs=**  RndMeth=Zero  SaturateOnIntegerOverflow=on
  Multi2 : Product  Inputs=**  RndMeth=Zero  SaturateOnIntegerOverflow=on
  Sum : Sum  Inputs=|++
  Speed : Outport
  wires:
  Data Type Conversion1/1 -> Speed/1
  Data Type Conversion4/1 -> Delay1/1
  Velocity/1 -> Multi2/1  "VelocityRaw"
  Delay1/1 -> Multi1/2  "VelocityFilteredPrevious"
  Multi2/1 -> Sum/1
  Sum/1 -> Data Type Conversion1/1, Data Type Conversion4/1  "VelocityFiltered"
  Multi1/1 -> Sum/2
  Ks/1 -> Add/1, Multi2/2
  Constant6/1 -> Add/2
  Add/1 -> Multi1/1

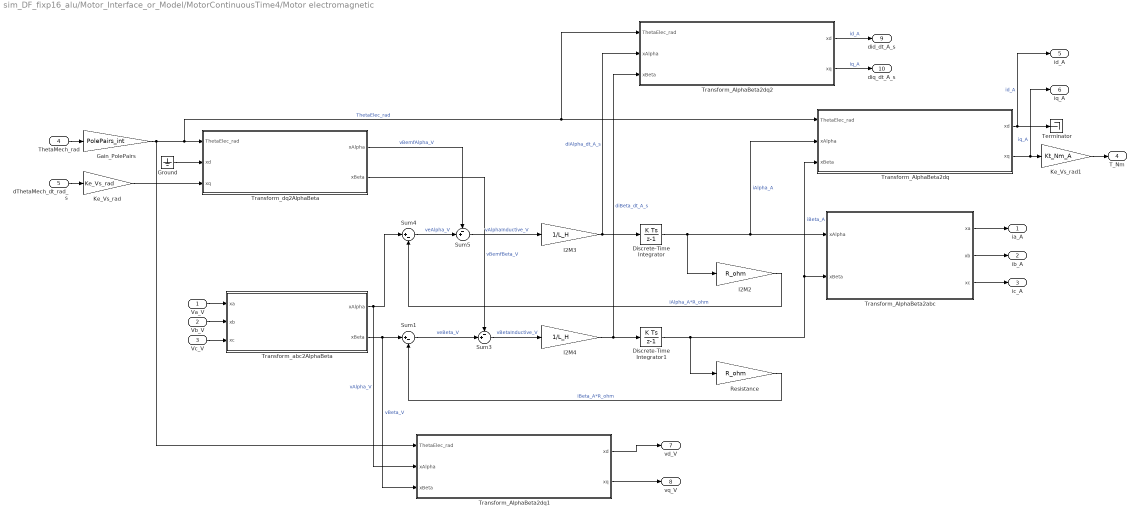
== system sim_DF_fixp16_alu/Motor_Interface_or_Model/MotorContinuousTime4/Motor electromagnetic ==
  Va_V : Inport
  Vb_V : Inport  Port=2
  Vc_V : Inport  Port=3
  ThetaMech_rad : Inport  Port=4
  dThetaMech_dt_rad_s : Inport  Port=5
  " Gain_PolePairs" : Gain  Gain=PolePairs_int
  Discrete-Time Integrator : DiscreteIntegrator  SampleTime=-1  ICPrevOutput=DiscIntNeverNeededParam  ICPrevScaledInput=DiscIntNeverNeededParam
  Discrete-Time Integrator1 : DiscreteIntegrator  SampleTime=-1  ICPrevOutput=DiscIntNeverNeededParam  ICPrevScaledInput=DiscIntNeverNeededParam
  Ground : Ground
  I2M2 : Gain  Gain=R_ohm
  I2M3 : Gain  Gain=1/L_H
  I2M4 : Gain  Gain=1/L_H
  Ke_Vs_rad : Gain  Gain=Ke_Vs_rad
  Ke_Vs_rad1 : Gain  Gain=Kt_Nm_A
  Resistance : Gain  Gain=R_ohm
  Sum1 : Sum  Inputs=|+-
  Sum3 : Sum  Inputs=-+|
  Sum4 : Sum  Inputs=|+-
  Sum5 : Sum  Inputs=-+|
  Terminator : Terminator
  Transform_AlphaBeta2abc : Subsystem  mask(Transform_AlphaBeta2abc){}
      mask help:
      | Transformation from equivalent Alpha-Beta 2-phase stator-based values to original 3-phase stator coil values.
      | Scaling chosen so peak values remain the same.
      mask Help:
      | Transformation from equivalent Alpha-Beta 2-phase stator-based values to original 3-phase stator coil values.
      | Scaling chosen so peak values remain the same.
      | Transformation equations:
      | 
      | xa = xAlpha
      | xb = -0.5*xAlpha + 0.5*sqrt(3)*xBeta
      | xc = -0.5*xAlpha - 0.5*sqrt(3)*xBeta
      mask Display:
      | port_label('output', 1, 'xa')
      | port_label('output', 2, 'xb')
      | port_label('output', 3, 'xc')
      | port_label('input', 1, 'xAlpha')
      | port_label('input', 2, 'xBeta')
      | disp ('xa=xAlpha\nxb=-0.5*xAlpha+0.5*sqrt(3)*xBeta\nxc=-0.5*xAlpha-0.5*sqrt(3)*xBeta');
  Transform_AlphaBeta2dq : Subsystem  mask(Transform_AlphaBeta2dq){}
      mask help: Transformation from Alpha-Beta to dq alignment.
      mask Help:
      | Transformation from Alpha-Beta to dq alignment.
      | Just a rotation, no change in magnitude:
      | 
      | xd = xAlpha*cos(Theta_rad) + xBeta*sin(Theta_rad)
      | xq = -xAlpha*sin(Theta_rad) + xBeta*cos(Theta_rad)
      mask Display:
      | port_label('output', 1, 'xd')
      | port_label('output', 2, 'xq')
      | port_label('input', 1, 'ThetaElec_rad')
      | port_label('input', 2, 'xAlpha')
      | port_label('input', 3, 'xBeta')
      | disp('xd=xAlpha*cos(Theta_rad)+xBeta*sin(Theta_rad)\nxq=-xAlpha*sin(Theta_rad)+xBeta*cos(Theta_rad)')
  Transform_AlphaBeta2dq1 : Subsystem  mask(Transform_AlphaBeta2dq){}
      mask help: Transformation from Alpha-Beta to dq alignment.
      mask Help:
      | Transformation from Alpha-Beta to dq alignment.
      | Just a rotation, no change in magnitude:
      | 
      | xd = xAlpha*cos(Theta_rad) + xBeta*sin(Theta_rad)
      | xq = -xAlpha*sin(Theta_rad) + xBeta*cos(Theta_rad)
      mask Display:
      | port_label('output', 1, 'xd')
      | port_label('output', 2, 'xq')
      | port_label('input', 1, 'ThetaElec_rad')
      | port_label('input', 2, 'xAlpha')
      | port_label('input', 3, 'xBeta')
      | disp('xd=xAlpha*cos(Theta_rad)+xBeta*sin(Theta_rad)\nxq=-xAlpha*sin(Theta_rad)+xBeta*cos(Theta_rad)')
  Transform_AlphaBeta2dq2 : Subsystem  mask(Transform_AlphaBeta2dq){}
      mask help: Transformation from Alpha-Beta to dq alignment.
      mask Help:
      | Transformation from Alpha-Beta to dq alignment.
      | Just a rotation, no change in magnitude:
      | 
      | xd = xAlpha*cos(Theta_rad) + xBeta*sin(Theta_rad)
      | xq = -xAlpha*sin(Theta_rad) + xBeta*cos(Theta_rad)
      mask Display:
      | port_label('output', 1, 'xd')
      | port_label('output', 2, 'xq')
      | port_label('input', 1, 'ThetaElec_rad')
      | port_label('input', 2, 'xAlpha')
      | port_label('input', 3, 'xBeta')
      | disp('xd=xAlpha*cos(Theta_rad)+xBeta*sin(Theta_rad)\nxq=-xAlpha*sin(Theta_rad)+xBeta*cos(Theta_rad)')
  Transform_abc2AlphaBeta : Subsystem  mask(Transform_abc_AlphaBeta){}
      mask help:
      | Transformation from 3-phase stator coil values to equivalent 2-phase values.
      | Scaling chosen so peak values remain the same.
      mask Help:
      | Transformation from 3-phase stator coil values to equivalent 2-phase values.
      | Scaling chosen so peak values remain the same.
      | Transformation equations:
      | 
      | xAlpha = 2/3*(xa - 0.5*xb - 0.5*xc)
      | xBeta = 2/3*(sqrt(3)/2*xb - sqrt(3)/2*xc)
      mask Display:
      | port_label('output', 1, 'xAlpha')
      | port_label('output', 2, 'xBeta')
      | port_label('input', 1, 'xa')
      | port_label('input', 2, 'xb')
      | port_label('input', 3, 'xc')
      | disp ('xAlpha=2/3*(xa-0.5*xb-0.5*xc)\nxBeta=2/3*(sqrt(3)/2*xb-sqrt(3)/2*xc)');
  Transform_dq2AlphaBeta : Subsystem  mask(Transform_dq_AlphaBeta){}
      mask help: Transformation from dq to AlphaBeta alignment.
      mask Help:
      | Transformation from dq to AlphaBeta alignment.
      | Just a rotation, no change in magnitude:
      | 
      | xAlpha = xd*cos(Theta_rad) - xq*sin(Theta_rad)
      | xBeta  = xd*sin(Theta_rad) + xq*cos(Theta_rad)
      mask Display:
      | port_label('output', 1, 'xAlpha')
      | port_label('output', 2, 'xBeta')
      | port_label('input', 1, 'ThetaElec_rad')
      | port_label('input', 2, 'xd')
      | port_label('input', 3, 'xq')
      | disp ('xAlpha=xd*cos(Theta_rad)-xq*sin(Theta_rad)\nxBeta=xd*sin(Theta_rad)+xq*cos(Theta_rad)');
  ia_A : Outport
  ib_A : Outport  Port=2
  ic_A : Outport  Port=3
  T_Nm : Outport  Port=4
  id_A : Outport  Port=5
  iq_A : Outport  Port=6
  vd_V : Outport  Port=7
  vq_V : Outport  Port=8
  did_dt_A_s : Outport  Port=9
  diq_dt_A_s : Outport  Port=10
  wires:
  ThetaMech_rad/1 -> " Gain_PolePairs"/1
  dThetaMech_dt_rad_s/1 -> Ke_Vs_rad/1
  Vb_V/1 -> Transform_abc2AlphaBeta/2(xb)
  Va_V/1 -> Transform_abc2AlphaBeta/1(xa)
  Vc_V/1 -> Transform_abc2AlphaBeta/3(xc)
  Transform_abc2AlphaBeta/1(xAlpha) -> Transform_AlphaBeta2dq1/2(xAlpha), Sum4/1  "vAlpha_V"
  Sum4/1 -> Sum5/2  "veAlpha_V"
  Sum3/1 -> I2M4/1  "vBetaInductive_V"
  " Gain_PolePairs"/1 -> Transform_AlphaBeta2dq1/1(ThetaElec_rad), Transform_AlphaBeta2dq2/1(ThetaElec_rad), Transform_AlphaBeta2dq/1(ThetaElec_rad), Transform_dq2AlphaBeta/1(ThetaElec_rad)  "ThetaElec_rad"
  Ground/1 -> Transform_dq2AlphaBeta/2(xd)
  Ke_Vs_rad/1 -> Transform_dq2AlphaBeta/3(xq)
  Transform_dq2AlphaBeta/1(xAlpha) -> Sum5/1  "vBemfAlpha_V"
  Transform_dq2AlphaBeta/2(xBeta) -> Sum3/1  "vBemfBeta_V"
  I2M4/1 -> Discrete-Time Integrator1/1, Transform_AlphaBeta2dq2/3(xBeta)  "diBeta_dt_A_s"
  Resistance/1 -> Sum1/2  "iBeta_A*R_ohm"
  Discrete-Time Integrator/1 -> I2M2/1, Transform_AlphaBeta2dq/2(xAlpha), Transform_AlphaBeta2abc/1(xAlpha)  "iAlpha_A"
  I2M2/1 -> Sum4/2  "iAlpha_A*R_ohm"
  I2M3/1 -> Discrete-Time Integrator/1, Transform_AlphaBeta2dq2/2(xAlpha)  "diAlpha_dt_A_s"
  Transform_abc2AlphaBeta/2(xBeta) -> Transform_AlphaBeta2dq1/3(xBeta), Sum1/1  "vBeta_V"
  Sum1/1 -> Sum3/2  "veBeta_V"
  Discrete-Time Integrator1/1 -> Transform_AlphaBeta2dq/3(xBeta), Transform_AlphaBeta2abc/2(xBeta), Resistance/1  "iBeta_A"
  Sum5/1 -> I2M3/1  "vAlphaInductive_V"
  Transform_AlphaBeta2abc/1(xa) -> ia_A/1
  Transform_AlphaBeta2abc/3(xc) -> ic_A/1
  Transform_AlphaBeta2abc/2(xb) -> ib_A/1
  Transform_AlphaBeta2dq/1(xd) -> id_A/1, Terminator/1  "id_A"
  Transform_AlphaBeta2dq/2(xq) -> iq_A/1, Ke_Vs_rad1/1  "iq_A"
  Ke_Vs_rad1/1 -> T_Nm/1
  Transform_AlphaBeta2dq1/2(xq) -> vq_V/1
  Transform_AlphaBeta2dq1/1(xd) -> vd_V/1
  Transform_AlphaBeta2dq2/1(xd) -> did_dt_A_s/1  "id_A"
  Transform_AlphaBeta2dq2/2(xq) -> diq_dt_A_s/1  "iq_A"

== system sim_DF_fixp16_alu/Motor_Interface_or_Model/MotorContinuousTime4/Motor inertia ==
  TA_Nm : Inport
  TB_Nm : Inport  Port=2
  Discrete-Time Integrator : DiscreteIntegrator  SampleTime=-1  ICPrevOutput=DiscIntNeverNeededParam  ICPrevScaledInput=DiscIntNeverNeededParam
  Discrete-Time Integrator1 : DiscreteIntegrator  SampleTime=-1  ICPrevOutput=DiscIntNeverNeededParam  ICPrevScaledInput=DiscIntNeverNeededParam
  InvMotorInertia_1_kgm2 : Gain  Gain=1/J_kgm2
  Sum1 : Sum  Inputs=+-
  dTheta_dt_rad_s : Outport
  Theta_rad : Outport  Port=2
  wires:
  TB_Nm/1 -> Sum1/2
  TA_Nm/1 -> Sum1/1  "U_ist_uvw_V"
  InvMotorInertia_1_kgm2/1 -> Discrete-Time Integrator/1  "d2Theta_dt2_rad_s2"
  Discrete-Time Integrator/1 -> Discrete-Time Integrator1/1, dTheta_dt_rad_s/1  "dTheta_dt_rad_s"
  Sum1/1 -> InvMotorInertia_1_kgm2/1
  Discrete-Time Integrator1/1 -> Theta_rad/1  "Theta_rad"

== system sim_DF_fixp16_alu/Altera_Cyclone_V_SoC/Speed_Control/Fix_PI_Ctrl_Integ1/Fixed Saturate1 ==
  In1 : Inport
  limit : Inport  Port=2
  CmpLT : RelationalOperator  Operator=<  OutDataTypeStr=boolean  RndMeth=Nearest
  CmpLT1 : RelationalOperator  OutDataTypeStr=boolean  RndMeth=Nearest
  Constant : Constant  Value=0  OutDataTypeStr=Inherit: Inherit via back propagation
  Subtract : Sum  Inputs=+-  AccumDataTypeStr=int32
  Switch : Switch  Criteria=u2 ~= 0  Threshold=Position_PI_Limit  ZeroCross=off
  Switch1 : Switch  Criteria=u2 ~= 0  Threshold=I_max  ZeroCross=off
  Out1 : Outport
  wires:
  Subtract/1 -> CmpLT/2, Switch1/1
  Switch1/1 -> Out1/1
  Switch/1 -> Switch1/3
  CmpLT/1 -> Switch1/2
  In1/1 -> CmpLT/1, Switch/3, CmpLT1/1
  limit/1 -> Subtract/2, CmpLT1/2, Switch/1
  Constant/1 -> Subtract/1
  CmpLT1/1 -> Switch/2

== system sim_DF_fixp16_alu/Altera_Cyclone_V_SoC/Speed_Control/Fix_PI_Ctrl_Integ1/Fixed Saturate2 ==
  In1 : Inport
  limit : Inport  Port=2
  CmpLT : RelationalOperator  Operator=<  OutDataTypeStr=boolean  RndMeth=Nearest
  CmpLT1 : RelationalOperator  OutDataTypeStr=boolean  RndMeth=Nearest
  Constant : Constant  Value=0  OutDataTypeStr=Inherit: Inherit via back propagation
  Subtract : Sum  Inputs=+-  AccumDataTypeStr=int32
  Switch : Switch  Criteria=u2 ~= 0  Threshold=Position_PI_Limit  ZeroCross=off
  Switch1 : Switch  Criteria=u2 ~= 0  Threshold=I_max  ZeroCross=off
  Out1 : Outport
  wires:
  Subtract/1 -> CmpLT/2, Switch1/1
  Switch1/1 -> Out1/1
  Switch/1 -> Switch1/3
  CmpLT/1 -> Switch1/2
  In1/1 -> CmpLT/1, Switch/3, CmpLT1/1
  limit/1 -> Subtract/2, CmpLT1/2, Switch/1
  Constant/1 -> Subtract/1
  CmpLT1/1 -> Switch/2

== system sim_DF_fixp16_alu/Altera_Cyclone_V_SoC/Speed_Control/Fix_PI_Ctrl_Integ1/Fixed Saturate3 ==
  In1 : Inport
  limit : Inport  Port=2
  CmpLT : RelationalOperator  Operator=<  OutDataTypeStr=boolean  RndMeth=Nearest
  CmpLT1 : RelationalOperator  OutDataTypeStr=boolean  RndMeth=Nearest
  Constant : Constant  Value=0  OutDataTypeStr=Inherit: Inherit via back propagation
  Subtract : Sum  Inputs=+-  AccumDataTypeStr=int32
  Switch : Switch  Criteria=u2 ~= 0  Threshold=Position_PI_Limit  ZeroCross=off
  Switch1 : Switch  Criteria=u2 ~= 0  Threshold=I_max  ZeroCross=off
  Out1 : Outport
  wires:
  CmpLT1/1 -> Switch/2
  Constant/1 -> Subtract/1
  limit/1 -> Switch/1, CmpLT1/2, Subtract/2
  In1/1 -> CmpLT1/1, Switch/3, CmpLT/1
  CmpLT/1 -> Switch1/2
  Switch/1 -> Switch1/3
  Switch1/1 -> Out1/1
  Subtract/1 -> Switch1/1, CmpLT/2

== system sim_DF_fixp16_alu/Motor_Interface_or_Model/MotorContinuousTime4/Motor electromagnetic/Transform_AlphaBeta2abc ==
  note: Transformation from equivalent Alpha-Beta 2-phase stator-based values to original 3-phase stator coil values.
      | Scaling chosen so peak values remain the same.
      | Transformation equations:
      |
      | xa = xAlpha
      | xb = -0.5*xAlpha + 0.5*sqrt(3)*xBeta
      | xc = -0.5*xAlpha - 0.5*sqrt(3)*xBeta
  xAlpha : Inport
  xBeta : Inport  Port=2
  Gain1 : Gain  Gain=0.5
  Gain3 : Gain  Gain=sqrt(3)
  Gain5 : Gain  Gain=0.5
  Sum1 : Sum  Inputs=-+
  Sum2 : Sum  Inputs=--
  xa : Outport
  xb : Outport  Port=2
  xc : Outport  Port=3
  wires:
  Gain5/1 -> xb/1
  Sum1/1 -> Gain5/1
  xAlpha/1 -> Sum2/1, Sum1/1, xa/1
  Gain3/1 -> Sum2/2, Sum1/2
  Gain1/1 -> xc/1
  Sum2/1 -> Gain1/1
  xBeta/1 -> Gain3/1

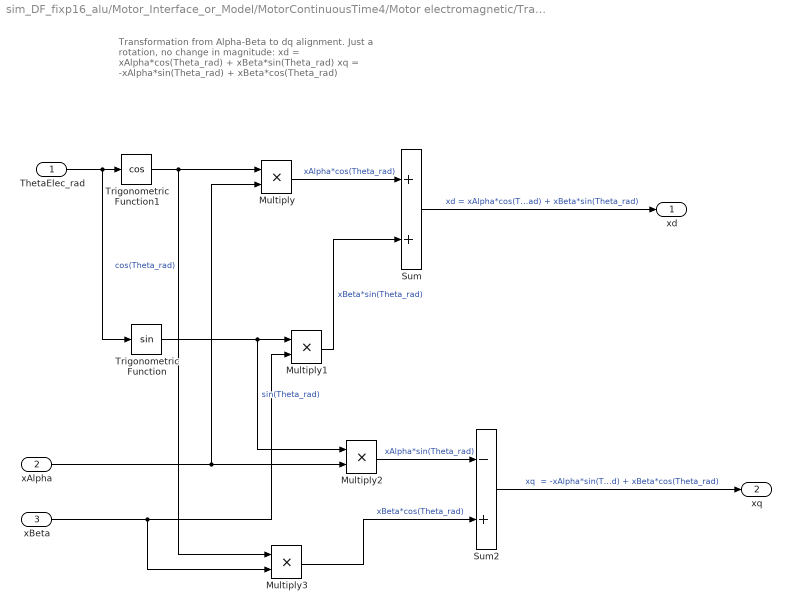
== system sim_DF_fixp16_alu/Motor_Interface_or_Model/MotorContinuousTime4/Motor electromagnetic/Transform_AlphaBeta2dq ==
  note: Transformation from Alpha-Beta to dq alignment.
      | Just a rotation, no change in magnitude:
      |
      | xd = xAlpha*cos(Theta_rad) + xBeta*sin(Theta_rad)
      | xq = -xAlpha*sin(Theta_rad) + xBeta*cos(Theta_rad)
  ThetaElec_rad : Inport
  xAlpha : Inport  Port=2
  xBeta : Inport  Port=3
  Multiply{,1..3} (4 alike) : Product  Inputs=**
  Sum : Sum
  Sum2 : Sum  Inputs=-+
  Trigonometric Function : Trigonometry
  Trigonometric Function1 : Trigonometry  Operator=cos
  xd : Outport
  xq : Outport  Port=2
  wires:
  Sum/1 -> xd/1  "xd = xAlpha*cos(Theta_rad) + xBeta*sin(Theta_rad)"
  Sum2/1 -> xq/1  "xq  = -xAlpha*sin(Theta_rad) + xBeta*cos(Theta_rad)"
  Multiply3/1 -> Sum2/2  "xBeta*cos(Theta_rad)"
  Multiply2/1 -> Sum2/1  "xAlpha*sin(Theta_rad)"
  Multiply1/1 -> Sum/2  "xBeta*sin(Theta_rad)"
  xBeta/1 -> Multiply1/2, Multiply3/2
  Trigonometric Function/1 -> Multiply1/1, Multiply2/1  "sin(Theta_rad)"
  Multiply/1 -> Sum/1  "xAlpha*cos(Theta_rad)"
  xAlpha/1 -> Multiply/2, Multiply2/2
  Trigonometric Function1/1 -> Multiply/1, Multiply3/1  "cos(Theta_rad)"
  ThetaElec_rad/1 -> Trigonometric Function1/1, Trigonometric Function/1

== system sim_DF_fixp16_alu/Motor_Interface_or_Model/MotorContinuousTime4/Motor electromagnetic/Transform_AlphaBeta2dq1 ==
  note: Transformation from Alpha-Beta to dq alignment.
      | Just a rotation, no change in magnitude:
      |
      | xd = xAlpha*cos(Theta_rad) + xBeta*sin(Theta_rad)
      | xq = -xAlpha*sin(Theta_rad) + xBeta*cos(Theta_rad)
  ThetaElec_rad : Inport
  xAlpha : Inport  Port=2
  xBeta : Inport  Port=3
  Multiply{,1..3} (4 alike) : Product  Inputs=**
  Sum : Sum
  Sum2 : Sum  Inputs=-+
  Trigonometric Function : Trigonometry
  Trigonometric Function1 : Trigonometry  Operator=cos
  xd : Outport
  xq : Outport  Port=2
  wires:
  Sum/1 -> xd/1  "xd = xAlpha*cos(Theta_rad) + xBeta*sin(Theta_rad)"
  Sum2/1 -> xq/1  "xq  = -xAlpha*sin(Theta_rad) + xBeta*cos(Theta_rad)"
  Multiply3/1 -> Sum2/2  "xBeta*cos(Theta_rad)"
  Multiply2/1 -> Sum2/1  "xAlpha*sin(Theta_rad)"
  Multiply1/1 -> Sum/2  "xBeta*sin(Theta_rad)"
  xBeta/1 -> Multiply1/2, Multiply3/2
  Trigonometric Function/1 -> Multiply1/1, Multiply2/1  "sin(Theta_rad)"
  Multiply/1 -> Sum/1  "xAlpha*cos(Theta_rad)"
  xAlpha/1 -> Multiply/2, Multiply2/2
  Trigonometric Function1/1 -> Multiply/1, Multiply3/1  "cos(Theta_rad)"
  ThetaElec_rad/1 -> Trigonometric Function1/1, Trigonometric Function/1

== system sim_DF_fixp16_alu/Motor_Interface_or_Model/MotorContinuousTime4/Motor electromagnetic/Transform_AlphaBeta2dq2 ==
  note: Transformation from Alpha-Beta to dq alignment.
      | Just a rotation, no change in magnitude:
      |
      | xd = xAlpha*cos(Theta_rad) + xBeta*sin(Theta_rad)
      | xq = -xAlpha*sin(Theta_rad) + xBeta*cos(Theta_rad)
  ThetaElec_rad : Inport
  xAlpha : Inport  Port=2
  xBeta : Inport  Port=3
  Multiply{,1..3} (4 alike) : Product  Inputs=**
  Sum : Sum
  Sum2 : Sum  Inputs=-+
  Trigonometric Function : Trigonometry
  Trigonometric Function1 : Trigonometry  Operator=cos
  xd : Outport
  xq : Outport  Port=2
  wires:
  ThetaElec_rad/1 -> Trigonometric Function/1, Trigonometric Function1/1
  Trigonometric Function1/1 -> Multiply3/1, Multiply/1  "cos(Theta_rad)"
  xAlpha/1 -> Multiply2/2, Multiply/2
  Multiply/1 -> Sum/1  "xAlpha*cos(Theta_rad)"
  Trigonometric Function/1 -> Multiply2/1, Multiply1/1  "sin(Theta_rad)"
  xBeta/1 -> Multiply3/2, Multiply1/2
  Multiply1/1 -> Sum/2  "xBeta*sin(Theta_rad)"
  Multiply2/1 -> Sum2/1  "xAlpha*sin(Theta_rad)"
  Multiply3/1 -> Sum2/2  "xBeta*cos(Theta_rad)"
  Sum2/1 -> xq/1  "xq  = -xAlpha*sin(Theta_rad) + xBeta*cos(Theta_rad)"
  Sum/1 -> xd/1  "xd = xAlpha*cos(Theta_rad) + xBeta*sin(Theta_rad)"

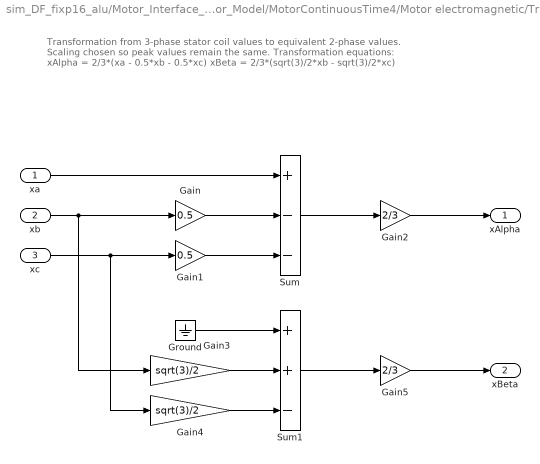
== system sim_DF_fixp16_alu/Motor_Interface_or_Model/MotorContinuousTime4/Motor electromagnetic/Transform_abc2AlphaBeta ==
  note: Transformation from 3-phase stator coil values to equivalent 2-phase values.
      | Scaling chosen so peak values remain the same.
      | Transformation equations:
      |
      | xAlpha = 2/3*(xa - 0.5*xb - 0.5*xc)
      | xBeta = 2/3*(sqrt(3)/2*xb - sqrt(3)/2*xc)
  xa : Inport
  xb : Inport  Port=2
  xc : Inport  Port=3
  Gain : Gain  Gain=0.5
  Gain1 : Gain  Gain=0.5
  Gain2 : Gain  Gain=2/3
  Gain3 : Gain  Gain=sqrt(3)/2
  Gain4 : Gain  Gain=sqrt(3)/2
  Gain5 : Gain  Gain=2/3
  Ground : Ground
  Sum : Sum  Inputs=+--
  Sum1 : Sum  Inputs=++-
  xAlpha : Outport
  xBeta : Outport  Port=2
  wires:
  xa/1 -> Sum/1
  xb/1 -> Gain3/1, Gain/1
  Gain/1 -> Sum/2
  xc/1 -> Gain4/1, Gain1/1
  Gain1/1 -> Sum/3
  Sum/1 -> Gain2/1
  Gain2/1 -> xAlpha/1
  Gain3/1 -> Sum1/2
  Gain4/1 -> Sum1/3
  Sum1/1 -> Gain5/1
  Gain5/1 -> xBeta/1
  Ground/1 -> Sum1/1

== system sim_DF_fixp16_alu/Motor_Interface_or_Model/MotorContinuousTime4/Motor electromagnetic/Transform_dq2AlphaBeta ==
  note: Transformation from dq to AlphaBeta alignment.
      | Just a rotation, no change in magnitude:
      |
      | xAlpha = xd*cos(Theta_rad) - xq*sin(Theta_rad)
      | xBeta  = xd*sin(Theta_rad) + xq*cos(Theta_rad)
  ThetaElec_rad : Inport
  xd : Inport  Port=2
  xq : Inport  Port=3
  Multiply{,1..3} (4 alike) : Product  Inputs=**
  Sum : Sum  Inputs=+-
  Sum2 : Sum
  Trigonometric Function : Trigonometry
  Trigonometric Function1 : Trigonometry  Operator=cos
  xAlpha : Outport
  xBeta : Outport  Port=2
  wires:
  ThetaElec_rad/1 -> Trigonometric Function/1, Trigonometric Function1/1
  Trigonometric Function1/1 -> Multiply3/1, Multiply/1  "cos(Theta_rad)"
  xd/1 -> Multiply2/2, Multiply/2
  Multiply/1 -> Sum/1  "xd*cos(Theta_rad)"
  Trigonometric Function/1 -> Multiply2/1, Multiply1/1  "sin(Theta_rad)"
  xq/1 -> Multiply3/2, Multiply1/2
  Multiply1/1 -> Sum/2  "xq*sin(Theta_rad)"
  Multiply2/1 -> Sum2/1  "xd*sin(Theta_rad)"
  Multiply3/1 -> Sum2/2  "xq*cos(Theta_rad)"
  Sum2/1 -> xBeta/1  "xBeta  = xd*sin(Theta_rad) + xq*cos(Theta_rad)"
  Sum/1 -> xAlpha/1  "xAlpha = xd*cos(Theta_rad) - xq*sin(Theta_rad)"

== matlab function sim_DF_fixp16_alu/Altera_Cyclone_V_SoC/Field_Oriented_Control/Motor_Interface ==
  data: pwm_max input; u_a input; u_b input; ru_out output; rv_out output; rw_out output
% Motor interface
function [ru_out, rv_out, rw_out] = fcn(pwm_max, u_a, u_b)

% Flag the functions that don't need to generate runtime code
coder.extrinsic('pathhelper', 'fullfile', 'strcat');

% Set up library paths
Root = strcat(pathhelper,'\mclib');
SrcPath = coder.const(fullfile(Root));
coder.cinclude('svm.h');
coder.updateBuildInfo('addSourceFiles','svm.c');
coder.updateBuildInfo('addSourcePaths',SrcPath);
coder.updateBuildInfo('addIncludePaths',SrcPath);

ru_out = uint16(0);
rv_out = uint16(0);
rw_out = uint16(0);

% Run motor control at the required update rate
coder.ceval('svm_interface',...
    pwm_max,...
    u_a,...
    u_b,...
    coder.wref(ru_out),...
    coder.wref(rv_out),...
    coder.wref(rw_out));
